simulink model "Inga"  (R2025a)
settings: Solver=VariableStepAuto  StartTime=0.0  StopTime=25  MaxStep=20e-3  RelTol=1e-3
InitFcn:
  | % A modell előkészítése futtatásra
  | 
  | % Modellparaméterek
  | g = 9.81;       % N/kg
  | rho_L = 1.2;	% kg/m^3
  | 
  | L = 1;
  | m = 2;
  | B = 0.5;        % Nms/rad
  | c_W = 0.47;
  | 
  | D = 0.1;
  | A = D^2*pi/4;
  | 
  | J = m*L^2;
  | 
  | % Kezdeti értékek
  | phi_0 = deg2rad(45);
  | omega_0 = 2;
settings Model: Creator=Szalay  LastModifiedBy=Szalay

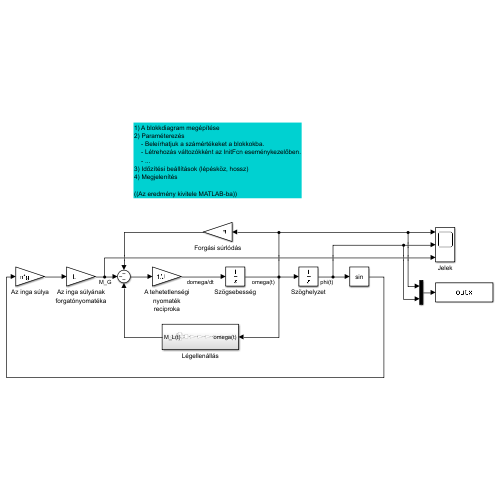
[thumbnail: Simulink's stored preview of the top-level diagram]
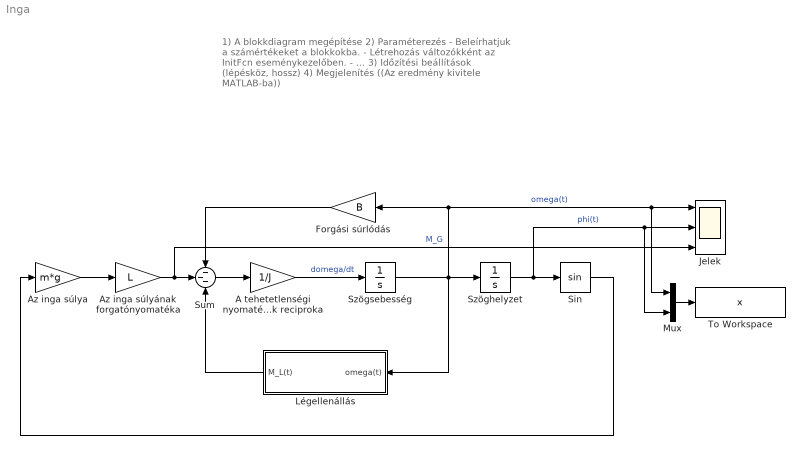
== system Inga ==
  note: 1) A blokkdiagram megépítése
      | 2) Paraméterezés
      |     - Beleírhatjuk a számértékeket a blokkokba.
      |     - Létrehozás változókként az InitFcn eseménykezelőben.
      |     - ...
      | 3) Időzítési beállítások (lépésköz, hossz)
      | 4) Megjelenítés
      |
      | ((Az eredmény kivitele MATLAB-ba))
  A tehetetlenségi nyomaték reciproka : Gain  Gain=1/J
  Az inga súlya : Gain  Gain=m*g
  Az inga súlyának forgatónyomatéka : Gain  Gain=L
  Forgási súrlódás : Gain  Gain=B
  Jelek : Scope  NumInputPorts=3
      settings: ActiveDisplayYMinimum=-1.1381694481657854  ActiveDisplayYMaximum=1.2747772294788311
  Légellenállás : Subsystem
  Mux : Mux  Inputs=2
  Sin : Trigonometry
  Sum : Sum  Inputs=---
  Szöghelyzet : Integrator  InitialCondition=phi_0
  Szögsebesség : Integrator  InitialCondition=omega_0
  To Workspace : ToWorkspace  VariableName=x  SaveFormat=Timeseries  SampleTime=-1
  wires:
  Szögsebesség/1 -> Légellenállás/1(omega(t)), Forgási súrlódás/1, Mux/1, Jelek/1, Szöghelyzet/1  "omega(t)"
  A tehetetlenségi nyomaték reciproka/1 -> Szögsebesség/1  "domega/dt"
  Sum/1 -> A tehetetlenségi nyomaték reciproka/1
  Forgási súrlódás/1 -> Sum/1
  Légellenállás/1(M_L(t)) -> Sum/3
  Szöghelyzet/1 -> Mux/2, Jelek/2, Sin/1  "phi(t)"
  Az inga súlyának forgatónyomatéka/1 -> Jelek/3, Sum/2  "M_G"
  Az inga súlya/1 -> Az inga súlyának forgatónyomatéka/1
  Sin/1 -> Az inga súlya/1
  Mux/1 -> To Workspace/1

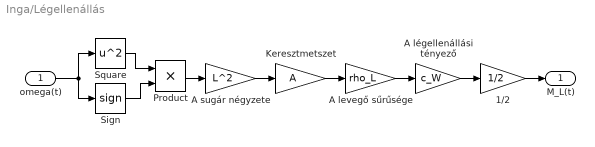
== system Inga/Légellenállás ==
  omega(t) : Inport
  1/2 : Gain  Gain=1/2
  A levegő sűrűsége : Gain  Gain=rho_L
  A légellenállási tényező : Gain  Gain=c_W
  A sugár négyzete : Gain  Gain=L^2
  Keresztmetszet : Gain  Gain=A
  Product : Product
  Sign : Signum
  Square : Math  Operator=square
  M_L(t) : Outport
  wires:
  Product/1 -> A sugár négyzete/1
  Sign/1 -> Product/2
  A sugár négyzete/1 -> Keresztmetszet/1
  A levegő sűrűsége/1 -> A légellenállási tényező/1
  omega(t)/1 -> Square/1, Sign/1
  Keresztmetszet/1 -> A levegő sűrűsége/1
  A légellenállási tényező/1 -> 1/2/1
  Square/1 -> Product/1
  1/2/1 -> M_L(t)/1
